simulink model "WorkstationModel"  (Simulink 8.6)
settings: Solver=VariableStepDiscrete  StartTime=0.0  StopTime=1000  RelTol=1e-3
settings Model: Creator=tsprock3  LastModifiedBy=tsprock3
settings DebuggingCC: FcnCallInpInsideContextMsg=EnableAllAsWarning  SimStateOlderReleaseMsg=warning
settings GRTTargetCC: CombineOutputUpdateFcns=on  GRTInterface=off

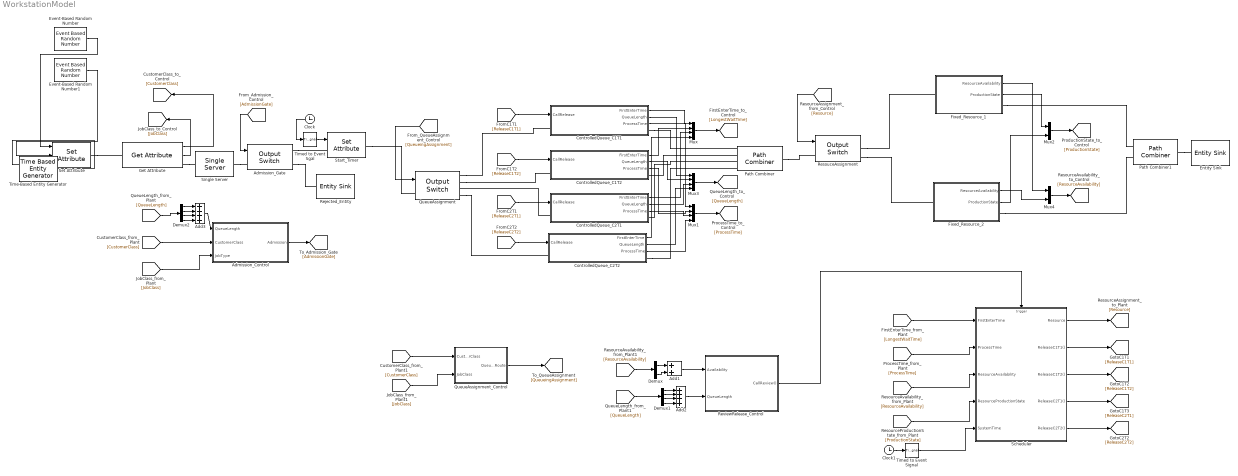
== system WorkstationModel ==
  Add1 : Sum
  Add2 : Sum  Inputs=++++
  Add3 : Sum  Inputs=++++
  Admission_Control : Stateflow chart  TreatAsAtomicUnit=on
  Admission_Gate : OutputSwitch  NumberOutputPorts=2  SwitchingCriterion=From signal port p
  Clock : Clock
  Clock1 : Clock
  ControlledQueue_C1T1 : Subsystem
  ControlledQueue_C1T2 : Subsystem
  ControlledQueue_C2T1 : Subsystem
  ControlledQueue_C2T2 : Subsystem
  Demux : Demux  Outputs=2
  Demux1 : Demux
  Demux2 : Demux
  Entity Sink : EntitySink
  Event-Based Random Number : EventBasedRandomNumber  Distribution=Arbitrary discrete  valueVecDisc=[1 2]  probVecDisc=[0.3 0.7]
  Event-Based Random Number1 : EventBasedRandomNumber  Distribution=Arbitrary discrete  valueVecDisc=[1 2]  probVecDisc=[.6 0.4]
  Fixed_Resource_1 : Subsystem
  Fixed_Resource_2 : Subsystem
  Get Attribute : GetAttribute  AttributeName=CustomerClass|JobClass  AttributeMissing=Error|Error  AttributeDefaultValue=1|1  AttributeTreatAsVector=1|1  AttributeSendTiming=After entity departure|After entity departure  EvaluatedDefaultAttributeValue={ [];[]}
      settings: OutputPortMap=o1,o2
  Mux : Mux
  Mux1 : Mux
  Mux2 : Mux  Inputs=2
  Mux3 : Mux
  Mux4 : Mux  Inputs=2
  Path Combiner : PathCombiner  NumberInputPorts=4
  Path Combiner1 : PathCombiner  NumberInputPorts=2
  QueueAssignment : OutputSwitch  NumberOutputPorts=4  SwitchingCriterion=From signal port p  EntityBufferOpt=on
  QueueAssignment_Control : Truth Table  TreatAsAtomicUnit=on
  Rejected_Entity : EntitySink
  ResouceAssignment : OutputSwitch  NumberOutputPorts=2  SwitchingCriterion=From signal port p  InitialConditionsOpt=on  EntityBufferOpt=on  StatLastDeparturePort=on
      settings: OutputPortMap=o3
  ReviewRelease_Control : Stateflow chart  TreatAsAtomicUnit=on
  Scheduler : MATLAB Function  TreatAsAtomicUnit=on
  Set Attribute : SetAttribute  AttributeName=CustomerClass|JobClass|ProcessTime  AttributeFrom=Signal port|Signal port|Dialog  AttributeValue=1|1|5  AttributeTreatAsVector=1|1|1  EvaluatedAttributeValue={ [];[];5}
      settings: InputPortMap=u0,u1
  Single Server : SingleServer  ServiceTime=0
  Start_Timer : SetAttribute  AttributeName=EnterTime  AttributeFrom=Signal port  EvaluatedAttributeValue={ []}
  Time-Based Entity Generator : TimeBasedEntityGenerator  Period=9
  Timed to Event Sgal : TimedToEventSignal
  Timed to Event Signal : TimedToEventSignal
  wires:
  ControlledQueue_C1T1/2(QueueLength) -> Mux3/1
  ControlledQueue_C1T2/2(QueueLength) -> Mux3/2
  ControlledQueue_C2T1/2(QueueLength) -> Mux3/3
  ControlledQueue_C2T2/2(QueueLength) -> Mux3/4
  Fixed_Resource_1/2(ProductionState) -> Mux2/1
  Mux2/1 -> [ProductionState]
  Mux/1 -> [LongestWaitTime]
  ControlledQueue_C1T1/1(FirstEnterTime) -> Mux/1
  ControlledQueue_C1T2/1(FirstEnterTime) -> Mux/2
  ControlledQueue_C2T1/1(FirstEnterTime) -> Mux/3
  ControlledQueue_C2T2/1(FirstEnterTime) -> Mux/4
  Mux1/1 -> [ProcessTime]
  ControlledQueue_C1T1/3(ProcessTime) -> Mux1/1
  ControlledQueue_C1T2/3(ProcessTime) -> Mux1/2
  ControlledQueue_C2T1/3(ProcessTime) -> Mux1/3
  ControlledQueue_C2T2/3(ProcessTime) -> Mux1/4
  [Resource] -> ResouceAssignment/1
  Event-Based Random Number/1 -> Set Attribute/1
  Event-Based Random Number1/1 -> Set Attribute/2
  Timed to Event Sgal/1 -> Start_Timer/1
  Clock/1 -> Timed to Event Sgal/1
  [LongestWaitTime] -> Scheduler/1(FirstEnterTime)
  [ReleaseC1T1] -> ControlledQueue_C1T1/1(CallRelease)
  [ReleaseC1T2] -> ControlledQueue_C1T2/1(CallRelease)
  [ReleaseC2T1] -> ControlledQueue_C2T1/1(CallRelease)
  [ReleaseC2T2] -> ControlledQueue_C2T2/1(CallRelease)
  QueueAssignment_Control/1(QueueRoute) -> [QueueingAssignment]
  [QueueingAssignment] -> QueueAssignment/1
  [AdmissionGate] -> Admission_Gate/1
  Get Attribute/1 -> [CustomerClass]
  Get Attribute/2 -> [JobClass]
  [CustomerClass] -> Admission_Control/2(CustomerClass)
  [JobClass] -> Admission_Control/3(JobType)
  [CustomerClass] -> QueueAssignment_Control/1(CustomerClass)
  [JobClass] -> QueueAssignment_Control/2(JobClass)
  Mux3/1 -> [QueueLength]
  [ResourceAvailability] -> Demux/1
  Demux/1 -> Add1/1
  Demux/2 -> Add1/2
  Mux4/1 -> [ResourceAvailability]
  Fixed_Resource_1/1(ResourceAvailability) -> Mux4/1
  Add1/1 -> ReviewRelease_Control/1(Availability)
  Fixed_Resource_2/2(ProductionState) -> Mux2/2
  Fixed_Resource_2/1(ResourceAvailability) -> Mux4/2
  ReviewRelease_Control/1(CallReview()) -> Scheduler/Trigger
  [ProcessTime] -> Scheduler/2(ProcessTime)
  [ResourceAvailability] -> Scheduler/3(ResourceAvailability)
  [ProductionState] -> Scheduler/4(ResourceProductionState)
  Scheduler/1(Resource) -> [Resource]
  Scheduler/2(ReleaseC1T1()) -> [ReleaseC1T1]
  Scheduler/3(ReleaseC1T2()) -> [ReleaseC1T2]
  Scheduler/4(ReleaseC2T1()) -> [ReleaseC2T1]
  Scheduler/5(ReleaseC2T2()) -> [ReleaseC2T2]
  [QueueLength] -> Demux2/1
  Demux2/1 -> Add3/1
  Demux2/2 -> Add3/2
  Demux2/3 -> Add3/3
  Add3/1 -> Admission_Control/1(QueueLength)
  Demux2/4 -> Add3/4
  Demux1/1 -> Add2/1
  Demux1/2 -> Add2/2
  Demux1/3 -> Add2/3
  Add2/1 -> ReviewRelease_Control/2(QueueLength)
  Demux1/4 -> Add2/4
  [QueueLength] -> Demux1/1
  Clock1/1 -> Timed to Event Signal/1
  Timed to Event Signal/1 -> Scheduler/5(SystemTime)
  Admission_Control/1(Admission) -> [AdmissionGate]
  connections:
  Fixed_Resource_1/RConn1 -- Path Combiner1/LConn1
  Admission_Gate/RConn1 -- Start_Timer/LConn1
  Single Server/RConn1 -- Admission_Gate/LConn1
  Get Attribute/RConn1 -- Single Server/LConn1
  Fixed_Resource_2/RConn1 -- Path Combiner1/LConn2
  Start_Timer/RConn1 -- QueueAssignment/LConn1
  QueueAssignment/RConn1 -- ControlledQueue_C1T1/LConn1
  QueueAssignment/RConn2 -- ControlledQueue_C1T2/LConn1
  ControlledQueue_C2T1/LConn1 -- QueueAssignment/RConn3
  QueueAssignment/RConn4 -- ControlledQueue_C2T2/LConn1
  ResouceAssignment/RConn1 -- Fixed_Resource_1/LConn1
  ResouceAssignment/RConn2 -- Fixed_Resource_2/LConn1
  Path Combiner/RConn1 -- ResouceAssignment/LConn1
  ControlledQueue_C1T1/RConn1 -- Path Combiner/LConn1
  ControlledQueue_C1T2/RConn1 -- Path Combiner/LConn2
  ControlledQueue_C2T1/RConn1 -- Path Combiner/LConn3
  ControlledQueue_C2T2/RConn1 -- Path Combiner/LConn4
  Path Combiner1/RConn1 -- Entity Sink/LConn1
  Time-Based Entity Generator/RConn1 -- Set Attribute/LConn1
  Set Attribute/RConn1 -- Get Attribute/LConn1
  Admission_Gate/RConn2 -- Rejected_Entity/LConn1

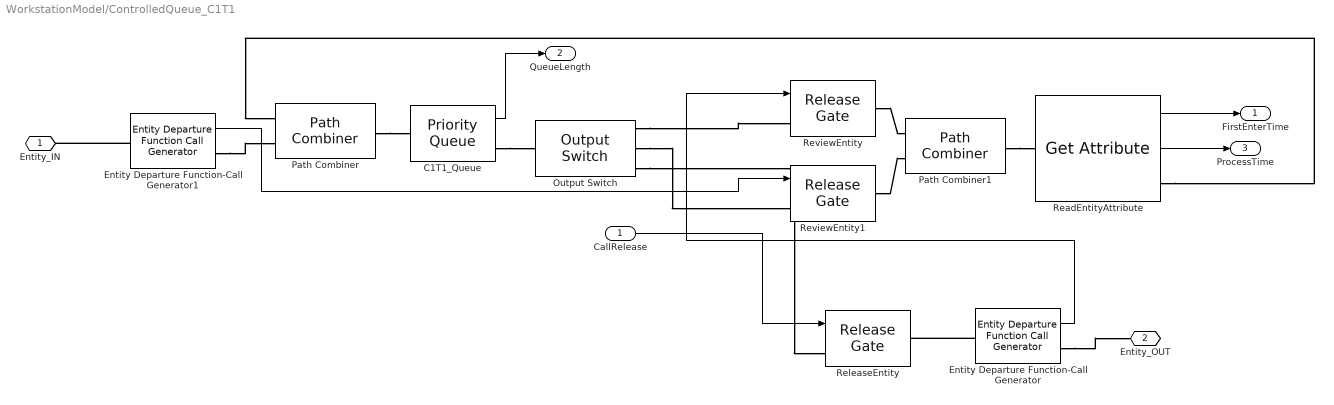
== system WorkstationModel/ControlledQueue_C1T1 ==
  CallRelease : Inport
  C1T1_Queue : PriorityQueue  Capacity=inf  SortingAttributeName=EnterTime  StatNumberInBlock=on
      settings: OutputPortMap=o1
  Entity Departure Function-Call Generator : EntityDepartureFunctionCallGenerator
  Entity Departure Function-Call Generator1 : EntityDepartureFunctionCallGenerator
  Output Switch : OutputSwitch
  Path Combiner : PathCombiner  NumberInputPorts=2
  Path Combiner1 : PathCombiner  NumberInputPorts=2
  ReadEntityAttribute : GetAttribute  AttributeName=EnterTime|ProcessTime  AttributeMissing=Error|Error  AttributeDefaultValue=1|1  AttributeTreatAsVector=1|1  AttributeSendTiming=After entity departure|After entity departure  EvaluatedDefaultAttributeValue={ [];[]}
      settings: OutputPortMap=o1,o2
  ReleaseEntity : ReleaseGate  OpenGateUpon=Function call from port fcn
  ReviewEntity : ReleaseGate  OpenGateUpon=Function call from port fcn  SignalEdgeOption=Either
  ReviewEntity1 : ReleaseGate  OpenGateUpon=Function call from port fcn  SignalEdgeOption=Either
  Entity_IN : PMIOPort  Port=1  Side=Left
  Entity_OUT : PMIOPort  Port=2  Side=Right
  FirstEnterTime : Outport
  QueueLength : Outport  Port=2
  ProcessTime : Outport  Port=3
  wires:
  C1T1_Queue/1 -> QueueLength/1
  ReadEntityAttribute/2 -> ProcessTime/1
  CallRelease/1 -> ReleaseEntity/1
  Entity Departure Function-Call Generator/1 -> ReviewEntity/1
  Entity Departure Function-Call Generator1/1 -> ReviewEntity1/1
  ReadEntityAttribute/1 -> FirstEnterTime/1
  connections:
  Path Combiner/RConn1 -- C1T1_Queue/LConn1
  C1T1_Queue/RConn1 -- Output Switch/LConn1
  ReadEntityAttribute/RConn1 -- Path Combiner/LConn1
  Entity Departure Function-Call Generator/LConn1 -- ReleaseEntity/RConn1
  Entity Departure Function-Call Generator/RConn1 -- Entity_OUT/RConn1
  Entity Departure Function-Call Generator1/LConn1 -- Entity_IN/RConn1
  Entity Departure Function-Call Generator1/RConn1 -- Path Combiner/LConn2
  Output Switch/RConn3 -- ReleaseEntity/LConn1
  Output Switch/RConn2 -- ReviewEntity1/LConn1
  Output Switch/RConn1 -- ReviewEntity/LConn1
  ReviewEntity/RConn1 -- Path Combiner1/LConn1
  ReviewEntity1/RConn1 -- Path Combiner1/LConn2
  Path Combiner1/RConn1 -- ReadEntityAttribute/LConn1

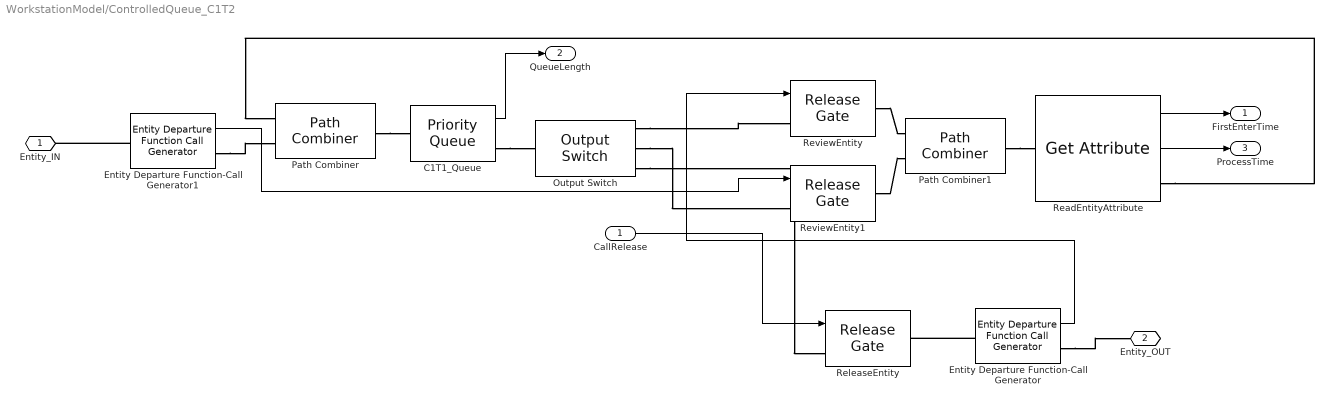
== system WorkstationModel/ControlledQueue_C1T2 ==
  CallRelease : Inport
  C1T1_Queue : PriorityQueue  Capacity=inf  SortingAttributeName=EnterTime  StatNumberInBlock=on
      settings: OutputPortMap=o1
  Entity Departure Function-Call Generator : EntityDepartureFunctionCallGenerator
  Entity Departure Function-Call Generator1 : EntityDepartureFunctionCallGenerator
  Output Switch : OutputSwitch
  Path Combiner : PathCombiner  NumberInputPorts=2
  Path Combiner1 : PathCombiner  NumberInputPorts=2
  ReadEntityAttribute : GetAttribute  AttributeName=EnterTime|ProcessTime  AttributeMissing=Error|Error  AttributeDefaultValue=1|1  AttributeTreatAsVector=1|1  AttributeSendTiming=After entity departure|After entity departure  EvaluatedDefaultAttributeValue={ [];[]}
      settings: OutputPortMap=o1,o2
  ReleaseEntity : ReleaseGate  OpenGateUpon=Function call from port fcn
  ReviewEntity : ReleaseGate  OpenGateUpon=Function call from port fcn  SignalEdgeOption=Either
  ReviewEntity1 : ReleaseGate  OpenGateUpon=Function call from port fcn  SignalEdgeOption=Either
  Entity_IN : PMIOPort  Port=1  Side=Left
  Entity_OUT : PMIOPort  Port=2  Side=Right
  FirstEnterTime : Outport
  QueueLength : Outport  Port=2
  ProcessTime : Outport  Port=3
  wires:
  ReadEntityAttribute/1 -> FirstEnterTime/1
  C1T1_Queue/1 -> QueueLength/1
  ReadEntityAttribute/2 -> ProcessTime/1
  CallRelease/1 -> ReleaseEntity/1
  Entity Departure Function-Call Generator/1 -> ReviewEntity/1
  Entity Departure Function-Call Generator1/1 -> ReviewEntity1/1
  connections:
  Path Combiner/RConn1 -- C1T1_Queue/LConn1
  C1T1_Queue/RConn1 -- Output Switch/LConn1
  ReadEntityAttribute/RConn1 -- Path Combiner/LConn1
  Entity Departure Function-Call Generator/LConn1 -- ReleaseEntity/RConn1
  Entity Departure Function-Call Generator/RConn1 -- Entity_OUT/RConn1
  Entity Departure Function-Call Generator1/LConn1 -- Entity_IN/RConn1
  Entity Departure Function-Call Generator1/RConn1 -- Path Combiner/LConn2
  Output Switch/RConn3 -- ReleaseEntity/LConn1
  Output Switch/RConn2 -- ReviewEntity1/LConn1
  Output Switch/RConn1 -- ReviewEntity/LConn1
  ReviewEntity/RConn1 -- Path Combiner1/LConn1
  ReviewEntity1/RConn1 -- Path Combiner1/LConn2
  Path Combiner1/RConn1 -- ReadEntityAttribute/LConn1

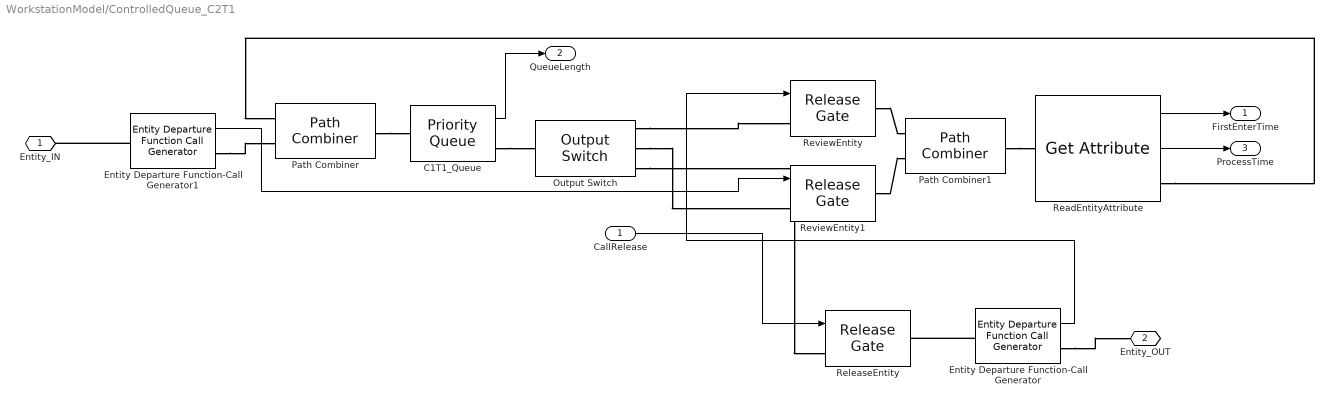
== system WorkstationModel/ControlledQueue_C2T1 ==
  CallRelease : Inport
  C1T1_Queue : PriorityQueue  Capacity=inf  SortingAttributeName=EnterTime  StatNumberInBlock=on
      settings: OutputPortMap=o1
  Entity Departure Function-Call Generator : EntityDepartureFunctionCallGenerator
  Entity Departure Function-Call Generator1 : EntityDepartureFunctionCallGenerator
  Output Switch : OutputSwitch
  Path Combiner : PathCombiner  NumberInputPorts=2
  Path Combiner1 : PathCombiner  NumberInputPorts=2
  ReadEntityAttribute : GetAttribute  AttributeName=EnterTime|ProcessTime  AttributeMissing=Error|Error  AttributeDefaultValue=1|1  AttributeTreatAsVector=1|1  AttributeSendTiming=After entity departure|After entity departure  EvaluatedDefaultAttributeValue={ [];[]}
      settings: OutputPortMap=o1,o2
  ReleaseEntity : ReleaseGate  OpenGateUpon=Function call from port fcn
  ReviewEntity : ReleaseGate  OpenGateUpon=Function call from port fcn  SignalEdgeOption=Either
  ReviewEntity1 : ReleaseGate  OpenGateUpon=Function call from port fcn  SignalEdgeOption=Either
  Entity_IN : PMIOPort  Port=1  Side=Left
  Entity_OUT : PMIOPort  Port=2  Side=Right
  FirstEnterTime : Outport
  QueueLength : Outport  Port=2
  ProcessTime : Outport  Port=3
  wires:
  ReadEntityAttribute/1 -> FirstEnterTime/1
  C1T1_Queue/1 -> QueueLength/1
  ReadEntityAttribute/2 -> ProcessTime/1
  CallRelease/1 -> ReleaseEntity/1
  Entity Departure Function-Call Generator/1 -> ReviewEntity/1
  Entity Departure Function-Call Generator1/1 -> ReviewEntity1/1
  connections:
  Path Combiner/RConn1 -- C1T1_Queue/LConn1
  C1T1_Queue/RConn1 -- Output Switch/LConn1
  ReadEntityAttribute/RConn1 -- Path Combiner/LConn1
  Entity Departure Function-Call Generator/LConn1 -- ReleaseEntity/RConn1
  Entity Departure Function-Call Generator/RConn1 -- Entity_OUT/RConn1
  Entity Departure Function-Call Generator1/LConn1 -- Entity_IN/RConn1
  Entity Departure Function-Call Generator1/RConn1 -- Path Combiner/LConn2
  Output Switch/RConn3 -- ReleaseEntity/LConn1
  Output Switch/RConn2 -- ReviewEntity1/LConn1
  Output Switch/RConn1 -- ReviewEntity/LConn1
  ReviewEntity/RConn1 -- Path Combiner1/LConn1
  ReviewEntity1/RConn1 -- Path Combiner1/LConn2
  Path Combiner1/RConn1 -- ReadEntityAttribute/LConn1

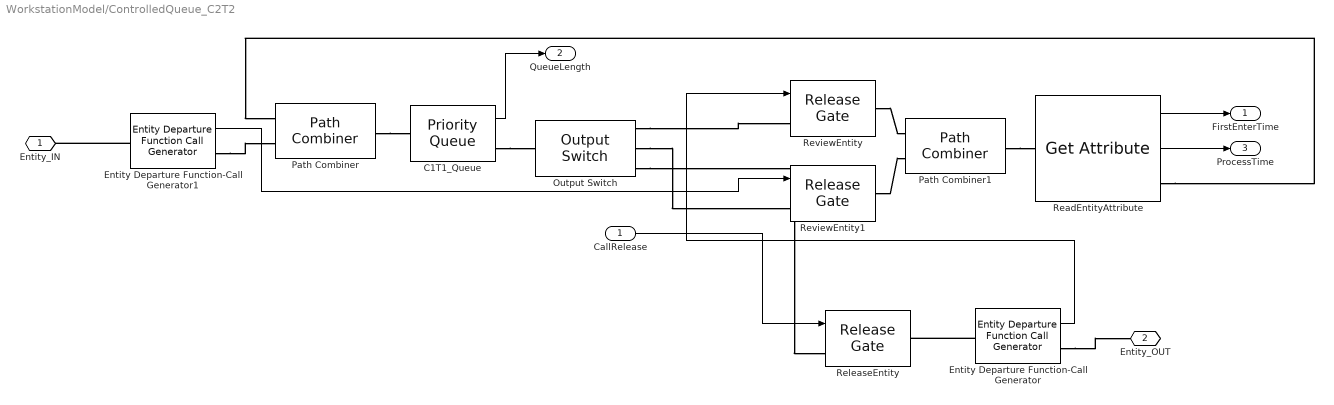
== system WorkstationModel/ControlledQueue_C2T2 ==
  CallRelease : Inport
  C1T1_Queue : PriorityQueue  Capacity=inf  SortingAttributeName=EnterTime  StatNumberInBlock=on
      settings: OutputPortMap=o1
  Entity Departure Function-Call Generator : EntityDepartureFunctionCallGenerator
  Entity Departure Function-Call Generator1 : EntityDepartureFunctionCallGenerator
  Output Switch : OutputSwitch
  Path Combiner : PathCombiner  NumberInputPorts=2
  Path Combiner1 : PathCombiner  NumberInputPorts=2
  ReadEntityAttribute : GetAttribute  AttributeName=EnterTime|ProcessTime  AttributeMissing=Error|Error  AttributeDefaultValue=1|1  AttributeTreatAsVector=1|1  AttributeSendTiming=After entity departure|After entity departure  EvaluatedDefaultAttributeValue={ [];[]}
      settings: OutputPortMap=o1,o2
  ReleaseEntity : ReleaseGate  OpenGateUpon=Function call from port fcn
  ReviewEntity : ReleaseGate  OpenGateUpon=Function call from port fcn  SignalEdgeOption=Either
  ReviewEntity1 : ReleaseGate  OpenGateUpon=Function call from port fcn  SignalEdgeOption=Either
  Entity_IN : PMIOPort  Port=1  Side=Left
  Entity_OUT : PMIOPort  Port=2  Side=Right
  FirstEnterTime : Outport
  QueueLength : Outport  Port=2
  ProcessTime : Outport  Port=3
  wires:
  ReadEntityAttribute/1 -> FirstEnterTime/1
  C1T1_Queue/1 -> QueueLength/1
  ReadEntityAttribute/2 -> ProcessTime/1
  CallRelease/1 -> ReleaseEntity/1
  Entity Departure Function-Call Generator/1 -> ReviewEntity/1
  Entity Departure Function-Call Generator1/1 -> ReviewEntity1/1
  connections:
  Path Combiner/RConn1 -- C1T1_Queue/LConn1
  C1T1_Queue/RConn1 -- Output Switch/LConn1
  ReadEntityAttribute/RConn1 -- Path Combiner/LConn1
  Entity Departure Function-Call Generator/LConn1 -- ReleaseEntity/RConn1
  Entity Departure Function-Call Generator/RConn1 -- Entity_OUT/RConn1
  Entity Departure Function-Call Generator1/LConn1 -- Entity_IN/RConn1
  Entity Departure Function-Call Generator1/RConn1 -- Path Combiner/LConn2
  Output Switch/RConn3 -- ReleaseEntity/LConn1
  Output Switch/RConn2 -- ReviewEntity1/LConn1
  Output Switch/RConn1 -- ReviewEntity/LConn1
  ReviewEntity/RConn1 -- Path Combiner1/LConn1
  ReviewEntity1/RConn1 -- Path Combiner1/LConn2
  Path Combiner1/RConn1 -- ReadEntityAttribute/LConn1

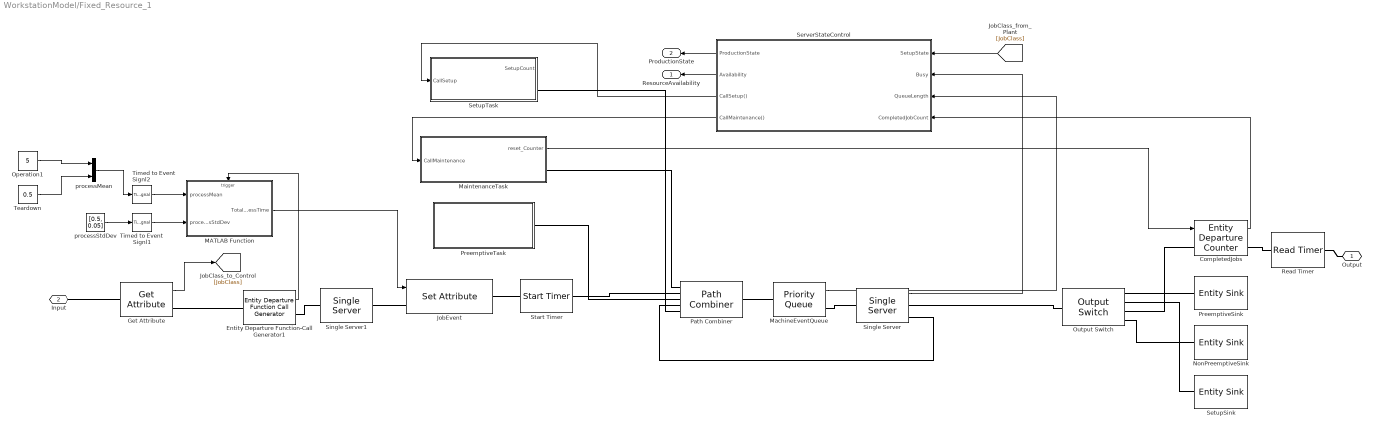
== system WorkstationModel/Fixed_Resource_1 ==
  CompletedJobs : EntityDepartureCounter  NumberDepartedToSignal=on  NumberDepartedToAttribute=off  CounterResetTypeOption=Function call from port fcn  SpecifyEventPriority=on
  Entity Departure Function-Call Generator1 : EntityDepartureFunctionCallGenerator
  Get Attribute : GetAttribute  AttributeName=JobClass  EvaluatedDefaultAttributeValue={ []}
      settings: OutputPortMap=o1
  JobEvent : SetAttribute  AttributeName=ServiceTime|PreemptiveEventClass  AttributeFrom=Signal port|Dialog  AttributeValue=1|3  AttributeTreatAsVector=1|1  EvaluatedAttributeValue={ [];3}
  MATLAB Function : MATLAB Function  TreatAsAtomicUnit=on
  MachineEventQueue : PriorityQueue  Capacity=inf  SortingAttributeName=PreemptiveEventClass  StatNumberInBlock=on
      settings: OutputPortMap=o1
  MaintenanceTask : Subsystem
  NonPreemptiveSink : EntitySink
  Operation1 : Constant  Value=5
  Output Switch : OutputSwitch  NumberOutputPorts=4  SwitchingCriterion=From attribute  AttributeName=PreemptiveEventClass
  Path Combiner : PathCombiner  NumberInputPorts=5
  PreemptiveSink : EntitySink
  PreemptiveTask : Subsystem
  Read Timer : ReadTimer
  ServerStateControl : Stateflow chart  TreatAsAtomicUnit=on
  SetupSink : EntitySink
  SetupTask : Subsystem
  Single Server : SingleServer  ServiceTimeFrom=Attribute  PermitPreemption=on  SortingAttributeName=PreemptiveEventClass  WriteToAttribute=on  ResidualAttributeName=ServiceTime  StatNumberInBlock=on
      settings: OutputPortMap=o1
  Single Server1 : SingleServer  ServiceTime=0
  Start Timer : StartTimer
  Teardown : Constant  Value=0.5
  Timed to Event Signl1 : TimedToEventSignal
  Timed to Event Signl2 : TimedToEventSignal
  processMean : Concatenate
  processStdDev : Constant  Value=[0.5, 0.05]
  Output : PMIOPort  Port=1  Side=Right
  Input : PMIOPort  Port=2  Side=Left
  ResourceAvailability : Outport
  ProductionState : Outport  Port=2
  wires:
  MATLAB Function/1(TotalProcessTime) -> JobEvent/1
  MaintenanceTask/1(reset_Counter) -> CompletedJobs/1
  Entity Departure Function-Call Generator1/1 -> MATLAB Function/Trigger
  processStdDev/1 -> Timed to Event Signl1/1
  Timed to Event Signl1/1 -> MATLAB Function/2(processStdDev)
  Timed to Event Signl2/1 -> MATLAB Function/1(processMean)
  processMean/1 -> Timed to Event Signl2/1
  Teardown/1 -> processMean/2
  Operation1/1 -> processMean/1
  ServerStateControl/3(CallSetup()) -> SetupTask/1(CallSetup)
  Single Server/1 -> ServerStateControl/2(Busy)
  MachineEventQueue/1 -> ServerStateControl/3(QueueLength)
  ServerStateControl/4(CallMaintenance()) -> MaintenanceTask/1(CallMaintenance)
  CompletedJobs/1 -> ServerStateControl/4(CompletedJobCount)
  ServerStateControl/1(ProductionState) -> ProductionState/1
  ServerStateControl/2(Availability) -> ResourceAvailability/1
  [JobClass] -> ServerStateControl/1(SetupState)
  Get Attribute/1 -> [JobClass]
  connections:
  MachineEventQueue/RConn1 -- Single Server/LConn1
  Path Combiner/RConn1 -- MachineEventQueue/LConn1
  Output Switch/RConn1 -- PreemptiveSink/LConn1
  Path Combiner/LConn4 -- Single Server/RConn2
  PreemptiveTask/RConn1 -- Path Combiner/LConn3
  MaintenanceTask/RConn1 -- Path Combiner/LConn1
  Entity Departure Function-Call Generator1/RConn1 -- Single Server1/LConn1
  Single Server1/RConn1 -- JobEvent/LConn1
  JobEvent/RConn1 -- Start Timer/LConn1
  Start Timer/RConn1 -- Path Combiner/LConn2
  CompletedJobs/RConn1 -- Read Timer/LConn1
  Read Timer/RConn1 -- Output/RConn1
  Single Server/RConn1 -- Output Switch/LConn1
  Path Combiner/LConn5 -- SetupTask/RConn1
  Get Attribute/RConn1 -- Entity Departure Function-Call Generator1/LConn1
  Input/RConn1 -- Get Attribute/LConn1
  CompletedJobs/LConn1 -- Output Switch/RConn3
  Output Switch/RConn2 -- SetupSink/LConn1
  NonPreemptiveSink/LConn1 -- Output Switch/RConn4

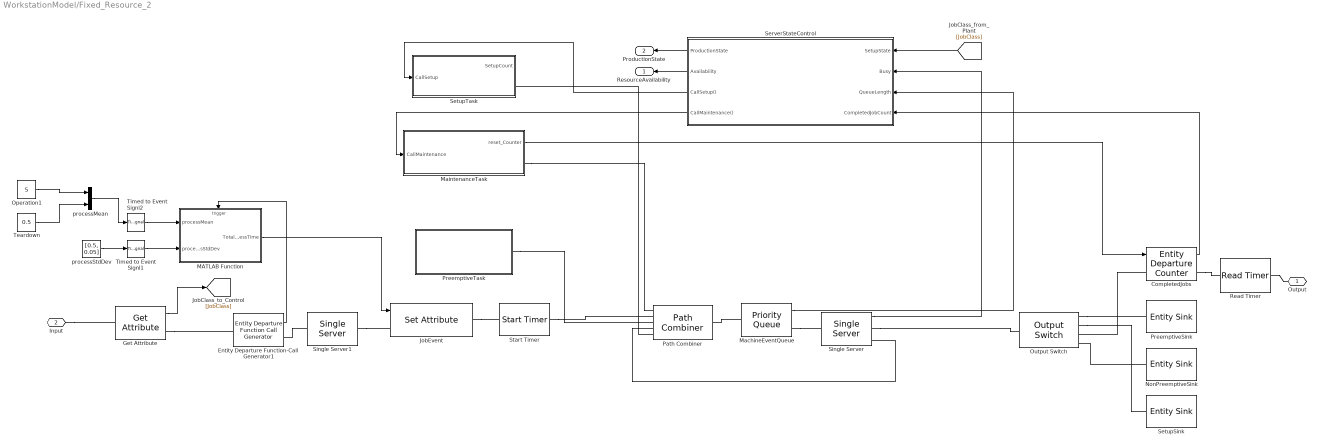
== system WorkstationModel/Fixed_Resource_2 ==
  CompletedJobs : EntityDepartureCounter  NumberDepartedToSignal=on  NumberDepartedToAttribute=off  CounterResetTypeOption=Function call from port fcn  SpecifyEventPriority=on
  Entity Departure Function-Call Generator1 : EntityDepartureFunctionCallGenerator
  Get Attribute : GetAttribute  AttributeName=JobClass  EvaluatedDefaultAttributeValue={ []}
      settings: OutputPortMap=o1
  JobEvent : SetAttribute  AttributeName=ServiceTime|PreemptiveEventClass  AttributeFrom=Signal port|Dialog  AttributeValue=1|3  AttributeTreatAsVector=1|1  EvaluatedAttributeValue={ [];3}
  MATLAB Function : MATLAB Function  TreatAsAtomicUnit=on
  MachineEventQueue : PriorityQueue  Capacity=inf  SortingAttributeName=PreemptiveEventClass  StatNumberInBlock=on
      settings: OutputPortMap=o1
  MaintenanceTask : Subsystem
  NonPreemptiveSink : EntitySink
  Operation1 : Constant  Value=5
  Output Switch : OutputSwitch  NumberOutputPorts=4  SwitchingCriterion=From attribute  AttributeName=PreemptiveEventClass
  Path Combiner : PathCombiner  NumberInputPorts=5
  PreemptiveSink : EntitySink
  PreemptiveTask : Subsystem
  Read Timer : ReadTimer
  ServerStateControl : Stateflow chart  TreatAsAtomicUnit=on
  SetupSink : EntitySink
  SetupTask : Subsystem
  Single Server : SingleServer  ServiceTimeFrom=Attribute  PermitPreemption=on  SortingAttributeName=PreemptiveEventClass  WriteToAttribute=on  ResidualAttributeName=ServiceTime  StatNumberInBlock=on
      settings: OutputPortMap=o1
  Single Server1 : SingleServer  ServiceTime=0
  Start Timer : StartTimer
  Teardown : Constant  Value=0.5
  Timed to Event Signl1 : TimedToEventSignal
  Timed to Event Signl2 : TimedToEventSignal
  processMean : Concatenate
  processStdDev : Constant  Value=[0.5, 0.05]
  Output : PMIOPort  Port=1  Side=Right
  Input : PMIOPort  Port=2  Side=Left
  ResourceAvailability : Outport
  ProductionState : Outport  Port=2
  wires:
  MATLAB Function/1(TotalProcessTime) -> JobEvent/1
  MaintenanceTask/1(reset_Counter) -> CompletedJobs/1
  Entity Departure Function-Call Generator1/1 -> MATLAB Function/Trigger
  processStdDev/1 -> Timed to Event Signl1/1
  Timed to Event Signl1/1 -> MATLAB Function/2(processStdDev)
  Timed to Event Signl2/1 -> MATLAB Function/1(processMean)
  processMean/1 -> Timed to Event Signl2/1
  Teardown/1 -> processMean/2
  Operation1/1 -> processMean/1
  ServerStateControl/3(CallSetup()) -> SetupTask/1(CallSetup)
  Single Server/1 -> ServerStateControl/2(Busy)
  MachineEventQueue/1 -> ServerStateControl/3(QueueLength)
  ServerStateControl/4(CallMaintenance()) -> MaintenanceTask/1(CallMaintenance)
  CompletedJobs/1 -> ServerStateControl/4(CompletedJobCount)
  ServerStateControl/1(ProductionState) -> ProductionState/1
  ServerStateControl/2(Availability) -> ResourceAvailability/1
  [JobClass] -> ServerStateControl/1(SetupState)
  Get Attribute/1 -> [JobClass]
  connections:
  MachineEventQueue/RConn1 -- Single Server/LConn1
  Path Combiner/RConn1 -- MachineEventQueue/LConn1
  Output Switch/RConn1 -- PreemptiveSink/LConn1
  Path Combiner/LConn4 -- Single Server/RConn2
  PreemptiveTask/RConn1 -- Path Combiner/LConn3
  MaintenanceTask/RConn1 -- Path Combiner/LConn1
  Entity Departure Function-Call Generator1/RConn1 -- Single Server1/LConn1
  Single Server1/RConn1 -- JobEvent/LConn1
  JobEvent/RConn1 -- Start Timer/LConn1
  Start Timer/RConn1 -- Path Combiner/LConn2
  CompletedJobs/RConn1 -- Read Timer/LConn1
  Read Timer/RConn1 -- Output/RConn1
  Single Server/RConn1 -- Output Switch/LConn1
  Path Combiner/LConn5 -- SetupTask/RConn1
  Get Attribute/RConn1 -- Entity Departure Function-Call Generator1/LConn1
  Input/RConn1 -- Get Attribute/LConn1
  CompletedJobs/LConn1 -- Output Switch/RConn3
  Output Switch/RConn2 -- SetupSink/LConn1
  NonPreemptiveSink/LConn1 -- Output Switch/RConn4

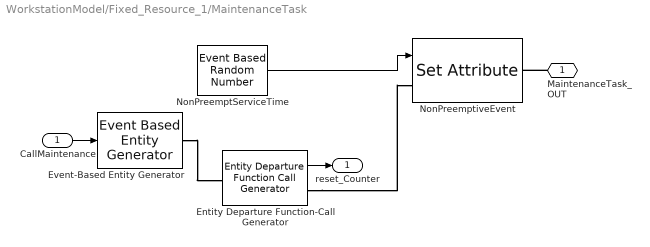
== system WorkstationModel/Fixed_Resource_1/MaintenanceTask ==
  CallMaintenance : Inport
  Entity Departure Function-Call Generator : EntityDepartureFunctionCallGenerator
  Event-Based Entity Generator : EventBasedEntityGenerator  GenerateEntitiesUpon=Function call from port fcn  GenerateEntityAtSimulationStart=off
  NonPreemptServiceTime : EventBasedRandomNumber  Seed=13927
  NonPreemptiveEvent : SetAttribute  AttributeName=ServiceTime|PreemptiveEventClass  AttributeFrom=Signal port|Dialog  AttributeValue=1|4  AttributeTreatAsVector=1|1  EvaluatedAttributeValue={ [];4}
  MaintenanceTask_OUT : PMIOPort  Port=1  Side=Right
  reset_Counter : Outport
  wires:
  NonPreemptServiceTime/1 -> NonPreemptiveEvent/1
  CallMaintenance/1 -> Event-Based Entity Generator/1
  Entity Departure Function-Call Generator/1 -> reset_Counter/1
  connections:
  Event-Based Entity Generator/RConn1 -- Entity Departure Function-Call Generator/LConn1
  Entity Departure Function-Call Generator/RConn1 -- NonPreemptiveEvent/LConn1
  MaintenanceTask_OUT/RConn1 -- NonPreemptiveEvent/RConn1

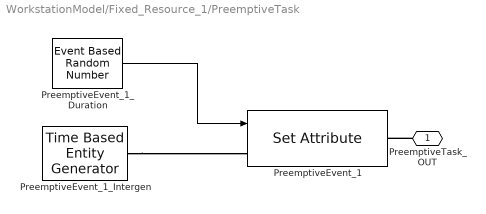
== system WorkstationModel/Fixed_Resource_1/PreemptiveTask ==
  PreemptiveEvent_1 : SetAttribute  AttributeName=ServiceTime|PreemptiveEventClass  AttributeFrom=Signal port|Dialog  AttributeValue=1|1  AttributeTreatAsVector=1|1  EvaluatedAttributeValue={ [];1}
  PreemptiveEvent_1_Duration : EventBasedRandomNumber  meanExp=3
  PreemptiveEvent_1_Intergen : TimeBasedEntityGenerator  Period=100  GenerateEntityAtSimulationStart=off
  PreemptiveTask_OUT : PMIOPort  Port=1  Side=Right
  wires:
  PreemptiveEvent_1_Duration/1 -> PreemptiveEvent_1/1
  connections:
  PreemptiveEvent_1_Intergen/RConn1 -- PreemptiveEvent_1/LConn1
  PreemptiveTask_OUT/RConn1 -- PreemptiveEvent_1/RConn1

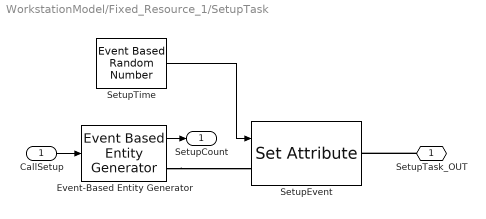
== system WorkstationModel/Fixed_Resource_1/SetupTask ==
  CallSetup : Inport
  Event-Based Entity Generator : EventBasedEntityGenerator  GenerateEntitiesUpon=Function call from port fcn  GenerateEntityAtSimulationStart=off  StatNumberDeparted=on
  SetupEvent : SetAttribute  AttributeName=ServiceTime|PreemptiveEventClass  AttributeFrom=Signal port|Dialog  AttributeValue=1|2  AttributeTreatAsVector=1|1  EvaluatedAttributeValue={ [];2}
  SetupTime : EventBasedRandomNumber  Seed=17144
  SetupTask_OUT : PMIOPort  Port=1  Side=Right
  SetupCount : Outport
  wires:
  SetupTime/1 -> SetupEvent/1
  CallSetup/1 -> Event-Based Entity Generator/1
  Event-Based Entity Generator/1 -> SetupCount/1
  connections:
  Event-Based Entity Generator/RConn1 -- SetupEvent/LConn1
  SetupTask_OUT/RConn1 -- SetupEvent/RConn1

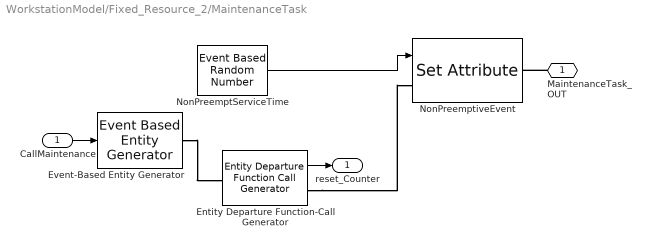
== system WorkstationModel/Fixed_Resource_2/MaintenanceTask ==
  CallMaintenance : Inport
  Entity Departure Function-Call Generator : EntityDepartureFunctionCallGenerator
  Event-Based Entity Generator : EventBasedEntityGenerator  GenerateEntitiesUpon=Function call from port fcn  GenerateEntityAtSimulationStart=off
  NonPreemptServiceTime : EventBasedRandomNumber  Seed=13927
  NonPreemptiveEvent : SetAttribute  AttributeName=ServiceTime|PreemptiveEventClass  AttributeFrom=Signal port|Dialog  AttributeValue=1|4  AttributeTreatAsVector=1|1  EvaluatedAttributeValue={ [];4}
  MaintenanceTask_OUT : PMIOPort  Port=1  Side=Right
  reset_Counter : Outport
  wires:
  NonPreemptServiceTime/1 -> NonPreemptiveEvent/1
  CallMaintenance/1 -> Event-Based Entity Generator/1
  Entity Departure Function-Call Generator/1 -> reset_Counter/1
  connections:
  Event-Based Entity Generator/RConn1 -- Entity Departure Function-Call Generator/LConn1
  Entity Departure Function-Call Generator/RConn1 -- NonPreemptiveEvent/LConn1
  MaintenanceTask_OUT/RConn1 -- NonPreemptiveEvent/RConn1

== system WorkstationModel/Fixed_Resource_2/PreemptiveTask ==
  PreemptiveEvent_1 : SetAttribute  AttributeName=ServiceTime|PreemptiveEventClass  AttributeFrom=Signal port|Dialog  AttributeValue=1|1  AttributeTreatAsVector=1|1  EvaluatedAttributeValue={ [];1}
  PreemptiveEvent_1_Duration : EventBasedRandomNumber  meanExp=3
  PreemptiveEvent_1_Intergen : TimeBasedEntityGenerator  Period=100  GenerateEntityAtSimulationStart=off
  PreemptiveTask_OUT : PMIOPort  Port=1  Side=Right
  wires:
  PreemptiveEvent_1_Duration/1 -> PreemptiveEvent_1/1
  connections:
  PreemptiveEvent_1_Intergen/RConn1 -- PreemptiveEvent_1/LConn1
  PreemptiveTask_OUT/RConn1 -- PreemptiveEvent_1/RConn1

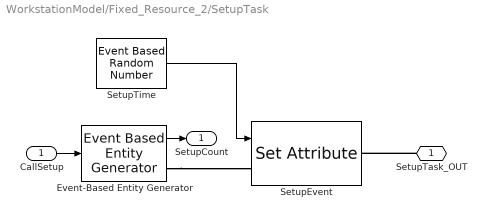
== system WorkstationModel/Fixed_Resource_2/SetupTask ==
  CallSetup : Inport
  Event-Based Entity Generator : EventBasedEntityGenerator  GenerateEntitiesUpon=Function call from port fcn  GenerateEntityAtSimulationStart=off  StatNumberDeparted=on
  SetupEvent : SetAttribute  AttributeName=ServiceTime|PreemptiveEventClass  AttributeFrom=Signal port|Dialog  AttributeValue=1|2  AttributeTreatAsVector=1|1  EvaluatedAttributeValue={ [];2}
  SetupTime : EventBasedRandomNumber  Seed=17144
  SetupTask_OUT : PMIOPort  Port=1  Side=Right
  SetupCount : Outport
  wires:
  SetupTime/1 -> SetupEvent/1
  CallSetup/1 -> Event-Based Entity Generator/1
  Event-Based Entity Generator/1 -> SetupCount/1
  connections:
  Event-Based Entity Generator/RConn1 -- SetupEvent/LConn1
  SetupTask_OUT/RConn1 -- SetupEvent/RConn1

== matlab function Fixed_Resource_1/MATLAB Function ==
  data: TotalProcessTime output double; processMean input double; processStdDev input double
  events: Arrival input FUNCTION_CALL_EVENT
function TotalProcessTime = fcn(processMean, processStdDev)
%#codegen

coder.extrinsic('normrnd');
TotalProcessTime = zeros(1,'double');

TotalProcessTime = sum(normrnd(processMean, processStdDev));

== matlab function Fixed_Resource_2/MATLAB Function ==
  data: TotalProcessTime output double; processMean input double; processStdDev input double
  events: Arrival input FUNCTION_CALL_EVENT
function TotalProcessTime = fcn(processMean, processStdDev)
%#codegen

coder.extrinsic('normrnd');
TotalProcessTime = zeros(1,'double');

TotalProcessTime = sum(normrnd(processMean, processStdDev));

== stateflow chart Fixed_Resource_2/ServerStateControl ==
  state ProductionState [parallel]
    settings: executionOrder=1
    state Type2
      entry: CallSetup;
      during: ProductionState =2;
    state Type1
      entry: CallSetup;
      during: ProductionState =1;
    (default) -> Type1
    Type2 -> Type1 : [SetupState ==1]
    Type1 -> Type2 : [SetupState ==2]
  state AvailabilityState [parallel]
    settings: executionOrder=2
    state Available
      en, du: Availability = 1;
    state Not_Available
      en, du: Availability =0;
    (default) -> Available
    Available -> Not_Available : [Busy ==1 || QueueLength >0]
    Not_Available -> Available : [Busy == 0 && QueueLength ==0]
  state MaintenanceState [parallel]
    settings: executionOrder=3
    state M0
    state M1
      en: CallMaintenance;
    (default) -> M0
    M0 -> M1 : [CompletedJobCount ==10]
    M1 -> M0 : [CompletedJobCount ==0]
  data: ProductionState output double; SetupState input double; Busy input double; QueueLength input double; Availability output double; CompletedJobCount input double
  events: CallSetup output FUNCTION_CALL_EVENT; CallMaintenance output FUNCTION_CALL_EVENT

== stateflow chart ReviewRelease_Control ==
  state CallReview_Control [parallel]
    settings: executionOrder=1
    state Queue [parallel]
      settings: executionOrder=1
      state Empty
      state NotEmpty
      (default) -> Empty
      NotEmpty -> Empty : [QueueLength ==0]
      Empty -> NotEmpty : [QueueLength >0]
    state Resource [parallel]
      settings: executionOrder=2
      state Available
      state Unavailable
      Available -> Unavailable : [Availability==0]
      Unavailable -> Available : [Availability >0]
      (default) -> Available
    state CallReview [parallel]
      settings: executionOrder=3
      state DoNothing
      state CallReview
        entry: CallReview;
      (default) -> DoNothing
      CallReview_Control.CallReview.CallReview -> DoNothing [order 1] : [in(Queue.Empty) || in(Resource.Unavailable)]
      DoNothing -> CallReview_Control.CallReview.CallReview : [in(Queue.NotEmpty) && in(Resource.Available)]
      CallReview_Control.CallReview.CallReview -> CallReview_Control.CallReview.CallReview [order 2] : [hasChanged(QueueLength) || hasChanged(Availability)]
  data: Availability input double; QueueLength input double
  events: CallReview output FUNCTION_CALL_EVENT

== stateflow chart Admission_Control ==
  state Reject_Task
    en: Admission = 2;
  state Admit_Task
    en: Admission = 1;
  (junction 80) -> Reject_Task [order 1] : [CustomerClass > 1]
  (junction 80) -> Admit_Task [order 2] : [CustomerClass == 1]
  (junction 81) -> (junction 80) [order 1] : [QueueLength>=10]
  (default) -> (junction 81)
  (junction 81) -> Admit_Task [order 2] : [QueueLength<10]
  data: QueueLength input double; CustomerClass input double; JobType input double; Admission output double

== matlab function QueueAssignment_Control ==
  data: CustomerClass input double; QueueRoute output double; JobClass input double
function QueueRoute = fcn(CustomerClass, JobClass)

aVarTruthTableCondition_1 = false;
aVarTruthTableCondition_2 = false;


% CustomerClass

aVarTruthTableCondition_1 = logical(CustomerClass==1);

% JobClass

aVarTruthTableCondition_2 = logical(JobClass==1);

if (aVarTruthTableCondition_1 && aVarTruthTableCondition_2)
    aFcnTruthTableAction_1();
elseif (aVarTruthTableCondition_1 && ~aVarTruthTableCondition_2)
    aFcnTruthTableAction_2();
elseif (~aVarTruthTableCondition_1 && aVarTruthTableCondition_2)
    aFcnTruthTableAction_3();
else % Default
    aFcnTruthTableAction_4();
end

function aFcnTruthTableAction_1()

% C1T1

QueueRoute = 1;

function aFcnTruthTableAction_2()

% C1T2

QueueRoute = 2;

function aFcnTruthTableAction_3()

% C2T1

QueueRoute = 3;

function aFcnTruthTableAction_4()

% C2T2

QueueRoute = 4;

== matlab function Scheduler ==
  data: FirstEnterTime input double; ProcessTime input double; ResourceAvailability input double; ResourceProductionState input double; Resource output double; SystemTime input double
  events: ServerAvailable input FUNCTION_CALL_EVENT; ReleaseC1T1 output FUNCTION_CALL_EVENT; ReleaseC1T2 output FUNCTION_CALL_EVENT; ReleaseC2T1 output FUNCTION_CALL_EVENT; ReleaseC2T2 output FUNCTION_CALL_EVENT
function Resource  = ScheduleControl(FirstEnterTime, ProcessTime, ResourceAvailability, ResourceProductionState, SystemTime)
%#codegen

NZ = find(ProcessTime);
%Release = [0 0 0 0];
ResourceAssignment = [1];
NextTask = 1;
Resource = 1;

if isempty(NZ) ==0
%% Create Schedule    
    
    quotedleadtime = [14 21 21 28]'; %[C1T1 C1T2 C2T1 C2T2]
    CostFactor = [3 3 6 6]';

    TotalDelay = SystemTime - FirstEnterTime + ProcessTime;
    TotalPenalty = CostFactor./(max(quotedleadtime-TotalDelay, 1)).^2;

    %Release job based on max penalty cost
    [Y, I] = sort(TotalPenalty(NZ));
    NextTask = NZ(I(1));

    %Insert some logic to assign resources meaningfully
    %Evaluate a flip between the top two tasks to minimize penalty cost or
    %set-ups
    
    
    
    %For now, 
    ResourceAssignment = find(ResourceAvailability);
    
    %This piece of code should pass a schedule to the bottom cell. TBD
    
%%  Execute Schedule

%Assign Resource to Task
    switch ResourceAssignment(1)
        case 1
            Resource = 1;
        case 2
            Resource = 2;
        otherwise
            Resource = 1;
    end

       
%Release a Job from a Queue
    switch NextTask
        case 1
            ReleaseC1T1;
        case 2
            ReleaseC1T2;
        case 3
            ReleaseC2T1;
        case 4
            ReleaseC2T2;
        otherwise
    end

end

== stateflow chart Fixed_Resource_1/ServerStateControl ==
  state ProductionState [parallel]
    settings: executionOrder=1
    state Type2
      entry: CallSetup;
      during: ProductionState =2;
    state Type1
      entry: CallSetup;
      during: ProductionState =1;
    (default) -> Type1
    Type1 -> Type2 : [SetupState ==2]
    Type2 -> Type1 : [SetupState ==1]
  state AvailabilityState [parallel]
    settings: executionOrder=2
    state Available
      en, du: Availability = 1;
    state Not_Available
      en, du: Availability =0;
    (default) -> Available
    Not_Available -> Available : [Busy == 0 && QueueLength ==0]
    Available -> Not_Available : [Busy ==1 || QueueLength >0]
  state MaintenanceState [parallel]
    settings: executionOrder=3
    state M0
    state M1
      en: CallMaintenance;
    (default) -> M0
    M1 -> M0 : [CompletedJobCount ==0]
    M0 -> M1 : [CompletedJobCount ==10]
  data: ProductionState output double; SetupState input double; Busy input double; QueueLength input double; Availability output double; CompletedJobCount input double
  events: CallSetup output FUNCTION_CALL_EVENT; CallMaintenance output FUNCTION_CALL_EVENT
